simulink model "DC_simulink"  (R2018a)
settings: Solver=VariableStepAuto  StartTime=0.0  StopTime=20  MaxStep=1e-3  RelTol=1e-3
settings Model: Creator=Aluno  LastModifiedBy=mpfva
settings SolverCC: ZeroCrossControl=DisableAll

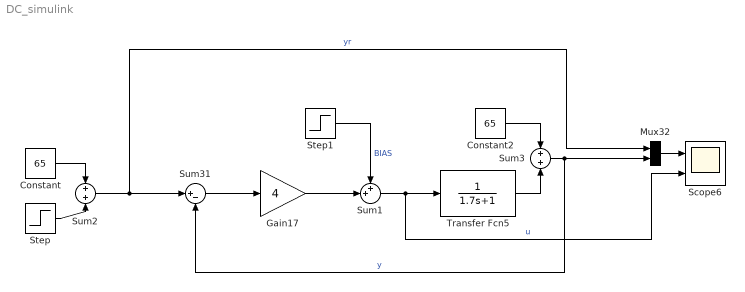
== system DC_simulink ==
  Constant : Constant  Value=65
  Constant2 : Constant  Value=65
  Gain17 : Gain  Gain=4
  Mux32 : Mux  Inputs=2
  Scope6 : Scope  NumInputPorts=2
  Step : Step  After=10  SampleTime=0
  Step1 : Step  After=10  SampleTime=0
  Sum1 : Sum  Inputs=++|
  Sum2 : Sum  Inputs=+|+
  Sum3 : Sum  Inputs=+|+
  Sum31 : Sum  Inputs=|+-
  Transfer Fcn5 : TransferFcn  Denominator=[1.7 1]
  wires:
  Sum2/1 -> Mux32/1, Sum31/1  "yr"
  Sum1/1 -> Scope6/2, Transfer Fcn5/1  "u"
  Sum31/1 -> Gain17/1
  Mux32/1 -> Scope6/1
  Gain17/1 -> Sum1/2
  Constant/1 -> Sum2/1
  Step/1 -> Sum2/2
  Constant2/1 -> Sum3/1
  Transfer Fcn5/1 -> Sum3/2
  Sum3/1 -> Mux32/2, Sum31/2  "y"
  Step1/1 -> Sum1/1  "BIAS"
